simulink library "tqd"  (R2021b)
settings: Solver=VariableStepAuto  StartTime=0.0  StopTime=10.0  RelTol=1e-3
undefined symbols (not defined in the file or in its folder): ATQD_APSDecReq_X_kph, ATQD_APSDecReq_Y_mps2, ATQD_APSDecReqCMD_X_kph, ATQD_APSDecReqTs_X_pct, ATQD_APSDecTimeGain_X_Deg, ATQD_APSDecTimeGain_Y_s, ATQD_APSReqLowSpd_X_Deg, ATQD_AutoHoldReleaseBPS_X_Deg, ATQD_AWDLoadTrqnsGain_X_kg, ATQD_AWDLoadTrqnsGain_Y_pct, ATQD_BOSEnBPSPosn_X_kph, ATQD_BOSMap_X_rpm, ATQD_BOSMap_Y_pct, ATQD_CreepBaseTqD_X_kph, ATQD_CreepBaseTqD_Y_Deg, ATQD_CreepBaseTqR_X_kph, ATQD_CreepBaseTqR_Y_Deg, ATQD_CreepBPSDisPosn_X_Deg, ATQD_CreepBPSDisPosnR_X_Deg, ATQD_CreepBPSEnPosn_X_Deg, ATQD_CreepBPSEnPosnR_X_Deg, ATQD_CreepDeltaTq_X_kph, ATQD_CreepIterm_X_kph, ATQD_CreepIterm_Y_kph, ATQD_CreepItermMaxLimit_X_pct, ATQD_CreepPreloadTime_X_kph, ATQD_CreepPreloadTq_X_kph, ATQD_CreepPreloadTq_Y_s, ATQD_CreepProtTq_X_Deg, ATQD_CreepPterm_X_kph, ATQD_CreepPterm_Y_kph, ATQD_ECOTqMapD_X_rpm, ATQD_ECOTqMapD_Y_pct, ATQD_EOPDTqMapDCon_X_rpm, ATQD_EOPDTqMapDCon_Y_Deg, ATQD_EstInitVehWeight_X_c, ATQD_LHMRollGenMapD_X_rpm, ATQD_LHMRollGenMapD_Y_rpm, ATQD_LHMTqMapD_X_rpm, ATQD_LHMTqMapD_Y_pct, ATQD_NL1TqMapD_X_rpm, ATQD_NL1TqMapD_Y_pct, ATQD_NOPDTqMapDCon_X_rpm, ATQD_NOPDTqMapDCon_Y_Deg, ATQD_NRMRrEDUSpRat_X_rpm, ATQD_NRMRrEDUSpRat_Y_Nm, ATQD_OPDHoldDownRelDelay_X_Deg, ATQD_OPDHoldEnSpd_X_Deg, ATQD_OPDHoldRelDetTime_X_Deg, ATQD_OPDHoldReleaseTq_X_Deg, ATQD_OrigPedTqLowLim_X_Deg, ATQD_OrigPedTqLowLim_Y_pct, ATQD_PedalMapClimbUpLim_X_rpm, ATQD_PedalMapClimbUpLim_Y_Deg, ATQD_PreLoadTq_X_s, ATQD_RollGenMapEL1_X_rpm, ATQD_RollGenMapEL1_Y_rpm, ATQD_SL1TqMapD_X_rpm, ATQD_SL1TqMapD_Y_pct, ATQD_SlideRegenTqGain_X_Gps ... (+487)
libraries: hcu_lib x83, simulink x73, tqr x1
(part 12 of 19)

== system tqd/TQD/TorqueDemand/TorqueModule/OPD Hold/Parking Requeest Backup ==
  VTQD_APSReq_enum : Inport
  VTQD_APSReqTimer_s : Inport  Port=2
  VTQD_ParkRequest_flg : Inport  Port=3
  task_time_s : Inport  Port=4
  VTQD_AutiHoldRelease_flg : Inport  Port=5
  AND : Logic  AllPortsSameDT=off  OutDataTypeStr=boolean
  AND1 : Logic  AllPortsSameDT=off  OutDataTypeStr=boolean
  AND3 : Logic  Inputs=3  AllPortsSameDT=off  OutDataTypeStr=boolean
  Constant1 : Constant  Value=KTQD_APSReqDelayTime_s
  Constant16 : Constant  OutDataTypeStr=uint8
  Constant17 : Constant  Value=TRUE  OutDataTypeStr=uint8
  Constant2 : Constant  Value=KTQD_APSReqDelayTime_s
  Constant3 : Constant  Value=KTQD_OPDHoldBrkSW_flg
  Constant4 : Constant  Value=KTQD_OPDHoldAllowPark_flg
  Constant5 : Constant  Value=KTQD_OPDHoldAllowPark_s
  Constant6 : Constant  Value=KTQD_OPDHoldAllowGearPSW_flg
  DelayEnable : hcu_lib/Basic_Blocks/DelayEnable
  Equal6 : RelationalOperator  Operator===  OutDataTypeStr=boolean  RndMeth=Simplest
  NOT : Logic  Operator=NOT  AllPortsSameDT=off  OutDataTypeStr=boolean
  OR : Logic  Operator=OR  AllPortsSameDT=off  OutDataTypeStr=boolean
  Relational Operator1 : RelationalOperator  OutDataTypeStr=boolean  RndMeth=Simplest
  Relational Operator6 : RelationalOperator  OutDataTypeStr=boolean  RndMeth=Simplest
  SR_Latch : hcu_lib/Basic_Blocks/SR_Latch
  Switch4 : Switch  Criteria=u2 > Threshold
  VTQD_ActParkRequest_flg : Outport
  VTQD_OPDHoldAllowPark_flg : Outport  Port=2
  wires:
  Constant3/1 -> AND3/2
  Constant1/1 -> Relational Operator6/2
  Equal6/1 -> AND3/1
  [VTQD_APSReq_enum] -> Equal6/1
  Relational Operator6/1 -> AND3/3
  [VTQD_ParkRequest_flg] -> Switch4/3
  Constant17/1 -> Switch4/1
  Constant16/1 -> Equal6/2
  Switch4/1 -> [VTQD_ActParkRequest_flg]  "VTQD_ActParkRequest_flg"
  [VTQD_APSReqTimer_s] -> Relational Operator6/1
  VTQD_APSReq_enum/1 -> [VTQD_APSReq_enum]
  VTQD_APSReqTimer_s/1 -> [VTQD_APSReqTimer_s]
  VTQD_ParkRequest_flg/1 -> [VTQD_ParkRequest_flg]
  [VTQD_ActParkRequest_flg] -> VTQD_ActParkRequest_flg/1
  Constant2/1 -> Relational Operator1/2
  [VTQD_APSReqTimer_s] -> Relational Operator1/1
  task_time_s/1 -> [task_time_s]
  AND/1 -> DelayEnable/1
  Relational Operator1/1 -> AND/1
  Constant4/1 -> AND/2
  Constant5/1 -> DelayEnable/2
  DelayEnable/1 -> SR_Latch/1
  [VTQD_AutiHoldRelease_flg] -> SR_Latch/2
  VTQD_AutiHoldRelease_flg/1 -> [VTQD_AutiHoldRelease_flg]
  SR_Latch/1 -> [VTQD_OPDHoldAllowPark_flg]  "VTQD_OPDHoldAllowPark_flg"
  OR/1 -> Switch4/2
  AND3/1 -> OR/1
  [task_time_s] -> DelayEnable/3
  [VTQD_OPDHoldAllowPark_flg] -> AND1/1
  AND1/1 -> OR/2
  NOT/1 -> AND1/2
  Constant6/1 -> NOT/1
  [VTQD_OPDHoldAllowPark_flg] -> VTQD_OPDHoldAllowPark_flg/1

== system tqd/TQD/TorqueDemand/TorqueModule/OPD Hold/Release Condition ==
  VVMC_EstSlope_Deg : Inport
  VTQD_VehActSpd_kph : Inport  Port=2
  VTQR_NoABSFEDUWhlTqReq_Nm : Inport  Port=3
  VTQR_NoABSREDUWhlTqReq_Nm : Inport  Port=4
  VTQD_ActBPSPosn_pct : Inport  Port=5
  task_time_s : Inport  Port=6
  VTQD_APSReqTimer_s : Inport  Port=7
  VTQD_LowIdleAccPedal_flg : Inport  Port=8
  VTQD_OPDHoldRgnOn2Off_flg : Inport  Port=9
  VTQD_ActAPSPosn_pct : Inport  Port=10
  VTQD_FrOPDHoldRelTqGain_Nm : Inport  Port=11
  VTQD_RrOPDHoldRelTqGain_Nm : Inport  Port=12
  AND : Logic  Inputs=3  AllPortsSameDT=off  OutDataTypeStr=boolean
  AND1 : Logic  AllPortsSameDT=off  OutDataTypeStr=boolean
  AND2 : Logic  AllPortsSameDT=off  OutDataTypeStr=boolean
  AND3 : Logic  AllPortsSameDT=off  OutDataTypeStr=boolean
  Add : Sum
  Add1 : Sum  Inputs=+-+
  Add6 : Sum
  Add7 : Sum
  Constant1 : Constant  Value=KTQD_APSRelDisTqDev_Nm
  Constant{5,10,23,30} (4 alike) : Constant  Value=ZERO_FLOAT
  Constant2 : Constant  Value=KTQD_OPDHoldDownEnTime_s
  Constant36 : Constant  Value=KTQD_OPDHoldRelDetSpd_kph
  Constant4 : Constant  Value=KTQD_OPDHoldRelTqGain_Nm
  Constant6 : Constant  Value=KTQD_OPDHoldDetRevSpd_kph
  Constant7 : Constant  Value=KTQD_OPDHoldLiftRevSpd_kph
  Constant8 : Constant  Value=KTQD_APSDecReqMaxTime_s
  Constant9 : Constant  Value=KTQD_OPDHoldRelTqGain_Nm
  Delay{,1..3} (4 alike) : Delay  DelayLength=1
  DelayEnable : hcu_lib/Basic_Blocks/DelayEnable
  DelayEnable1 : hcu_lib/Basic_Blocks/DelayEnable
  Detect Increase : simulink/Logic and Bit Operations/Detect Increase  vinit=0.0  OutDataTypeStr=boolean
  Detect Increase1 : simulink/Logic and Bit Operations/Detect Increase  vinit=0.0  OutDataTypeStr=boolean
  Detect Increase2 : simulink/Logic and Bit Operations/Detect Increase  vinit=0.0  OutDataTypeStr=boolean
  MTQD_AutoHoldReleaseBPS_Y_pct : Lookup_n-D  NumberOfTableDimensions=1  BreakpointsForDimension1=ATQD_AutoHoldReleaseBPS_X_Deg  Table=MTQD_AutoHoldReleaseBPS_Y_pct  InternalRulePriority=Speed  RndMeth=Simplest  InputSameDT=on
  MTQD_OPDHoldDownRelDelay_Y_s : Lookup_n-D  NumberOfTableDimensions=1  BreakpointsForDimension1=ATQD_OPDHoldDownRelDelay_X_Deg  Table=MTQD_OPDHoldDownRelDelay_Y_s  InternalRulePriority=Speed  RndMeth=Simplest  InputSameDT=on
  MTQD_OPDHoldRelDetTime_Y_s : Lookup_n-D  NumberOfTableDimensions=1  BreakpointsForDimension1=ATQD_OPDHoldRelDetTime_X_Deg  Table=MTQD_OPDHoldRelDetTime_Y_s  InternalRulePriority=Speed  RndMeth=Simplest  InputSameDT=on
  MTQD_OPDHoldReleaseTq_Y_Nm{,1..3} (4 alike) : Lookup_n-D  NumberOfTableDimensions=1  BreakpointsForDimension1=ATQD_OPDHoldReleaseTq_X_Deg  Table=MTQD_OPDHoldReleaseTq_Y_Nm  InternalRulePriority=Speed  RndMeth=Simplest  InputSameDT=on
  Max : MinMax  Function=max  Inputs=2
  Max1 : MinMax  Function=max  Inputs=2
  Max2 : MinMax  Function=max  Inputs=2
  NOT{,1..5} (6 alike) : Logic  Operator=NOT  AllPortsSameDT=off  OutDataTypeStr=boolean
  OR : Logic  Operator=OR  AllPortsSameDT=off  OutDataTypeStr=boolean
  OR1 : Logic  Operator=OR  AllPortsSameDT=off  OutDataTypeStr=boolean
  OR2 : Logic  Operator=OR  AllPortsSameDT=off  OutDataTypeStr=boolean
  OR3 : Logic  Operator=OR  Inputs=3  AllPortsSameDT=off  OutDataTypeStr=boolean
  Relational Operator : RelationalOperator  Operator=>  OutDataTypeStr=boolean  RndMeth=Simplest
  Relational Operator1 : RelationalOperator  Operator=<=  OutDataTypeStr=boolean  RndMeth=Simplest
  Relational Operator3 : RelationalOperator  Operator=<=  OutDataTypeStr=boolean  RndMeth=Simplest
  Relational Operator4 : RelationalOperator  OutDataTypeStr=boolean  RndMeth=Simplest
  Relational Operator5 : RelationalOperator  Operator=<  OutDataTypeStr=boolean  RndMeth=Simplest
  Relational Operator6 : RelationalOperator  Operator=>  OutDataTypeStr=boolean  RndMeth=Simplest
  Relational Operator7 : RelationalOperator  OutDataTypeStr=boolean  RndMeth=Simplest
  Relational Operator9 : RelationalOperator  OutDataTypeStr=boolean  RndMeth=Simplest
  Relay : Relay  OnSwitchValue=KTQD_OPDHoldGradeUp_Deg  OffSwitchValue=KTQD_OPDHoldGradeDown_Deg  OutDataTypeStr=boolean
  Relay1 : Relay  OnSwitchValue=KTQD_OPDHoldGradeUp_Deg  OffSwitchValue=KTQD_OPDHoldGradeDown_Deg  OutDataTypeStr=boolean
  SR_Latch : hcu_lib/Basic_Blocks/SR_Latch
  SR_Latch1 : hcu_lib/Basic_Blocks/SR_Latch
  Switch{,1..6} (7 alike) : Switch  Criteria=u2 > Threshold
  Terminator : Terminator
  VTQD_AutoHoldRelease_flg : Outport
  VTQD_OPDHoldEnRel_flg : Outport  Port=2
  VTQD_OPDHoldActRelTq_Nm : Outport  Port=3
  wires:
  VVMC_EstSlope_Deg/1 -> [VVMC_EstSlope_Deg]
  VTQD_VehActSpd_kph/1 -> [VTQD_VehActSpd_kph]
  VTQR_NoABSFEDUWhlTqReq_Nm/1 -> [VTQR_NoABSFEDUWhlTqReq_Nm]
  VTQR_NoABSREDUWhlTqReq_Nm/1 -> [VTQR_NoABSREDUWhlTqReq_Nm]
  VTQD_ActBPSPosn_pct/1 -> [VTQD_ActBPSPosn_pct]
  task_time_s/1 -> [task_time_s]
  [VTQD_AutoHoldRelease_flg] -> VTQD_AutoHoldRelease_flg/1
  [VTQD_OPDHoldEnRel_flg] -> VTQD_OPDHoldEnRel_flg/1
  VTQD_APSReqTimer_s/1 -> [VTQD_APSReqTimer_s]
  VTQD_LowIdleAccPedal_flg/1 -> [VTQD_LowIdleAccPedal_flg]
  VTQD_OPDHoldRgnOn2Off_flg/1 -> [VTQD_OPDHoldRgnOn2Off_flg]
  VTQD_ActAPSPosn_pct/1 -> Terminator/1
  VTQD_RrOPDHoldRelTqGain_Nm/1 -> [VTQD_RrOPDHoldRelTqGain_Nm]
  VTQD_FrOPDHoldRelTqGain_Nm/1 -> [VTQD_FrOPDHoldRelTqGain_Nm]
  SR_Latch/1 -> DelayEnable/1  "VTQD_OPDHoldEnRelLatch_flg"
  Detect Increase2/1 -> OR2/1
  Detect Increase1/1 -> SR_Latch1/1
  DelayEnable1/1 -> Switch1/1
  SR_Latch1/1 -> [VTQD_OPDHoldRelReverse_flg]  "VTQD_OPDHoldRelReverse_flg"
  MTQD_OPDHoldDownRelDelay_Y_s/1 -> [VTQD_OPDHoldDownRelDelay_s]  "VTQD_OPDHoldDownRelDelay_s"
  Constant4/1 -> Switch2/1
  [VVMC_EstSlope_Deg] -> MTQD_OPDHoldDownRelDelay_Y_s/1
  [task_time_s] -> DelayEnable1/3
  [VTQD_LowIdleAccPedal_flg] -> NOT2/1
  Constant30/1 -> Switch5/1
  NOT/1 -> AND/2
  [VVMC_EstSlope_Deg] -> Relay1/1
  Relay1/1 -> NOT3/1
  Constant2/1 -> Relational Operator1/2
  OR1/1 -> AND/3
  Switch1/1 -> Switch/3
  AND2/1 -> Switch1/3
  [VTQD_LowIdleAccPedal_flg] -> NOT1/1
  [VTQD_OPDHoldRgnOn2Off_flg] -> Switch/2
  Relational Operator/1 -> OR1/1
  Relational Operator1/1 -> AND/1
  [VTQD_OPDHoldRelDetTime_s] -> DelayEnable/2
  AND/1 -> OR/1
  [VVMC_EstSlope_Deg] -> Relay/1
  [VTQR_NoABSFEDUWhlTqReq_Nm] -> Add6/1
  [VTQR_NoABSREDUWhlTqReq_Nm] -> Add6/2
  [task_time_s] -> DelayEnable/3
  [VTQR_NoABSFEDUWhlTqReq_Nm] -> Add7/1
  [VTQD_ActBPSPosn_pct] -> Relational Operator/1
  Add1/1 -> Max1/1
  [VVMC_EstSlope_Deg] -> MTQD_OPDHoldReleaseTq_Y_Nm/1
  DelayEnable/1 -> [VTQD_OPDHoldEnRel_flg]  "VTQD_OPDHoldEnRel_flg"
  [VTQR_NoABSREDUWhlTqReq_Nm] -> Add7/2
  Max1/1 -> Relational Operator5/2
  [VTQD_VehActSpd_kph] -> Relational Operator9/1
  Relational Operator9/1 -> Switch5/2
  [VVMC_EstSlope_Deg] -> MTQD_AutoHoldReleaseBPS_Y_pct/1
  [VVMC_EstSlope_Deg] -> MTQD_OPDHoldRelDetTime_Y_s/1
  Switch5/1 -> [VTQD_OPDHoldRelDetTime_s]  "VTQD_OPDHoldRelDetTime_s"
  MTQD_AutoHoldReleaseBPS_Y_pct/1 -> Relational Operator/2  "VTQD_AutoHoldReleaseAPS_pct"
  OR/1 -> [VTQD_AutoHoldRelease_flg]  "VTQD_AutoHoldRelease_flg"
  MTQD_OPDHoldReleaseTq_Y_Nm/1 -> Switch6/3
  Relational Operator3/1 -> Detect Increase1/1
  [VTQD_OPDHoldDownRelDelay_s] -> DelayEnable1/2
  Delay3/1 -> Max2/1
  Max2/1 -> Switch6/1
  Constant6/1 -> Relational Operator3/2
  Detect Increase/1 -> OR3/1
  Add7/1 -> Relational Operator5/1  "VTQD_OPDHoldDisRelTq_Nm"
  Switch6/1 -> Add/2, Delay3/1  "VTQD_OPDHoldReleaseTq_Nm"
  [VVMC_EstSlope_Deg] -> MTQD_OPDHoldReleaseTq_Y_Nm3/1
  [VTQD_APSReqTimer_s] -> Delay/1
  NOT3/1 -> Switch1/2
  [VTQD_OPDHoldRelReverse_flg] -> Detect Increase2/1
  [VTQD_OPDHoldRelReverse_flg] -> Switch6/2
  Constant23/1 -> Max1/2
  [VTQD_LowIdleAccPedal_flg] -> NOT4/1
  MTQD_OPDHoldRelDetTime_Y_s/1 -> Switch5/3
  [VTQD_OPDHoldRelReverse_flg] -> Switch3/2
  Relational Operator4/1 -> SR_Latch/1  "VTQD_OPDHoldEnRelease_flg"
  Switch2/1 -> Add/1
  NOT5/1 -> AND2/2
  MTQD_OPDHoldReleaseTq_Y_Nm1/1 -> Switch4/3
  Relay/1 -> NOT/1
  Add/1 -> [VTQD_OPDHoldActRelTq_Nm], Relational Operator4/2  "VTQD_OPDHoldActRelTq_Nm"
  [VTQD_OPDHoldRelReverse_flg] -> Switch4/2
  Delay/1 -> Relational Operator1/1
  Constant8/1 -> Relational Operator7/2
  OR2/1 -> SR_Latch/2
  [VTQD_VehActSpd_kph] -> Relational Operator3/1
  Delay2/1 -> Max/1
  [VTQD_OPDHoldEnRel_flg] -> AND1/2
  AND1/1 -> Switch/1
  [VTQD_LowIdleAccPedal_flg] -> AND3/1
  [VTQD_LowIdleAccPedal_flg] -> NOT5/1
  Constant36/1 -> Relational Operator9/2
  NOT4/1 -> DelayEnable1/1
  [VTQD_APSReqTimer_s] -> Delay1/1
  Constant10/1 -> Switch3/3
  MTQD_OPDHoldReleaseTq_Y_Nm2/1 -> Max/2
  [VTQD_LowIdleAccPedal_flg] -> Detect Increase/1
  Add6/1 -> Relational Operator4/1  "VTQD_OPDHoldEnRelTq_flg"
  [VTQD_OPDHoldRelReverse_flg] -> Switch2/2
  Switch3/1 -> Add1/1
  [VVMC_EstSlope_Deg] -> MTQD_OPDHoldReleaseTq_Y_Nm1/1
  Relational Operator5/1 -> OR2/2  "VTQD_OPDHoldDisRelease_flg"
  MTQD_OPDHoldReleaseTq_Y_Nm3/1 -> Max2/2
  Delay1/1 -> Relational Operator7/1
  Relational Operator7/1 -> AND3/2
  Constant7/1 -> Relational Operator6/2
  Switch4/1 -> Delay2/1, Add1/3
  Constant5/1 -> Switch2/3
  AND3/1 -> OR3/3
  Constant9/1 -> Switch3/1
  Switch/1 -> OR/2
  NOT2/1 -> AND1/1
  [VTQD_VehActSpd_kph] -> Relational Operator6/1
  [VTQD_OPDHoldEnRel_flg] -> AND2/1
  Constant1/1 -> Add1/2
  NOT1/1 -> OR1/2
  Relational Operator6/1 -> OR3/2
  Max/1 -> Switch4/1
  [VVMC_EstSlope_Deg] -> MTQD_OPDHoldReleaseTq_Y_Nm2/1
  OR3/1 -> SR_Latch1/2
  [VTQD_OPDHoldActRelTq_Nm] -> VTQD_OPDHoldActRelTq_Nm/1

== system tqd/TQD/TorqueDemand/TorqueModule/OPD Hold/System Status ==
  VTQD_GearActualPosn_enum : Inport
  VINP_EPBSta_enum : Inport  Port=2
  VTQD_RegenMode_enum : Inport  Port=3
  VTQD_AutiHoldRelease_flg : Inport  Port=4
  VTQD_AntiBlockRrActDisTime_s : Inport  Port=5
  VTQD_RrAntiBlockAactive_flg : Inport  Port=6
  VTQD_ActBPSPosn_pct : Inport  Port=7
  VTQD_AntiBlockFrActDisTime_s : Inport  Port=8
  VTQD_FrAntiBlockAactive_flg : Inport  Port=9
  VVMC_ADASActive_flg : Inport  Port=10
  VPMM_PwrSta_enum : Inport  Port=11
  VVMC_CruzActive_flg : Inport  Port=12
  VTQD_VehActSpd_kph : Inport  Port=13
  VVMC_EstSlope_Deg : Inport  Port=14
  task_time_s : Inport  Port=15
  VINP_FrPTCSActive_flg : Inport  Port=16
  VINP_RrPTCSActive_flg : Inport  Port=17
  VINP_ESCActive_flg : Inport  Port=18
  VINP_ABSActive_flg : Inport  Port=19
  VVMC_APSActive_flg : Inport  Port=20
  AND{,3..6} (5 alike) : Logic  AllPortsSameDT=off  OutDataTypeStr=boolean
  AND1 : Logic  Inputs=4  AllPortsSameDT=off  OutDataTypeStr=boolean
  AND2 : Logic  Inputs=11  AllPortsSameDT=off  OutDataTypeStr=boolean
  Constant1 : Constant  Value=2  OutDataTypeStr=uint8
  Constant10 : Constant  Value=ENUM_GEARACTUALPOSN_R
  Constant11 : Constant  Value=ENUM_GEARACTUALPOSN_D
  Constant12 : Constant  Value=KTQD_R2DGradeUpLim_Deg
  Constant13 : Constant  Value=KTQD_R2DGradeLowLim_Deg
  Constant14 : Constant  Value=KTQD_R2DEnOPDHoldSpd_kph
  Constant15 : Constant  Value=KTQD_R2DEnOPDHSpdDelayTime_s
  Constant2 : Constant  Value=0  OutDataTypeStr=uint8
  Constant3 : Constant  Value=ENUM_EPBSTA_APPLIED
  Constant4 : Constant  Value=ENUM_GEARACTUALPOSN_P
  Constant40 : Constant  Value=ENUM_REGENLEVEL_OPD
  Constant44 : Constant  Value=ENUM_REGENLEVEL_OPD
  Constant45 : Constant  Value=ENUM_POWERSTA_READY
  Constant5 : Constant  Value=ENUM_GEARACTUALPOSN_D
  Constant6 : Constant  Value=KTQD_AutoHoldEnSpd_kph
  Constant7 : Constant  Value=ENUM_EPBSTA_APPLIED
  Constant8 : Constant  Value=ENUM_REGENLEVEL_OPD
  Constant9 : Constant  Value=ENUM_GEARACTUALPOSN_P
  Delay : Delay  DelayLength=1
  Delay2 : Delay  DelayLength=1
  Delay3 : Delay  DelayLength=1
  DelayEnable : hcu_lib/Basic_Blocks/DelayEnable
  Equal{1..2,5..6,8..9,11,30} (8 alike) : RelationalOperator  Operator===  OutDataTypeStr=boolean  RndMeth=Simplest
  Equal10 : RelationalOperator  Operator=~=  OutDataTypeStr=boolean  RndMeth=Simplest
  Equal3 : RelationalOperator  Operator=~=  OutDataTypeStr=boolean  RndMeth=Simplest
  Equal4 : RelationalOperator  Operator=~=  OutDataTypeStr=boolean  RndMeth=Simplest
  GreaterThan3 : RelationalOperator  Operator=>  OutDataTypeStr=boolean  RndMeth=Simplest
  NOT{,1..7} (8 alike) : Logic  Operator=NOT  AllPortsSameDT=off  OutDataTypeStr=boolean
  OR : Logic  Operator=OR  AllPortsSameDT=off  OutDataTypeStr=boolean
  OR1 : Logic  Operator=OR  AllPortsSameDT=off  OutDataTypeStr=boolean
  OR5 : Logic  Operator=OR  AllPortsSameDT=off  OutDataTypeStr=boolean
  Relational Operator : RelationalOperator  Operator=<=  OutDataTypeStr=boolean  RndMeth=Simplest
  Relational Operator1 : RelationalOperator  OutDataTypeStr=boolean  RndMeth=Simplest
  Relational Operator2 : RelationalOperator  OutDataTypeStr=boolean  RndMeth=Simplest
  Relational Operator3 : RelationalOperator  Operator=<=  OutDataTypeStr=boolean  RndMeth=Simplest
  SR_Latch3 : hcu_lib/Basic_Blocks/SR_Latch
  SR_Latch4 : hcu_lib/Basic_Blocks/SR_Latch
  Switch : Switch  Criteria=u2 > Threshold
  Unit Delay1 : UnitDelay  SampleTime=-1  HasFrameUpgradeWarning=on
  VTQD_APSStaSys_enum : Outport
  VTQD_OPDHoldDelayForP_flg : Outport  Port=2
  VTQD_OPDHoldRgnOn2Off_flg : Outport  Port=3
  wires:
  Switch/1 -> [VTQD_APSStaSys_enum]  "VTQD_APSStaSys_enum"
  Constant2/1 -> Switch/3
  AND2/1 -> Switch/2
  Constant1/1 -> Switch/1
  [VTQD_GearActualPosn_enum] -> Equal1/1
  Equal1/1 -> AND5/1
  AND5/1 -> [VTQD_OPDHoldDelayForP_flg]  "VTQD_OPDHoldDelayForP_flg"
  Equal10/1 -> AND5/2
  [VTQD_RegenMode_enum] -> Equal8/1
  OR5/1 -> [VTQD_AntiBlockEnOPDHold_flg]  "VTQD_AntiBlockEnOPDHold_flg"
  Equal8/1 -> OR5/2
  Constant40/1 -> Equal8/2
  Equal11/1 -> GreaterThan3/2, Unit Delay1/1
  SR_Latch3/1 -> [VTQD_OPDHoldRgnOn2Off_flg]  "VTQD_OPDHoldRgnOn2Off_flg"
  GreaterThan3/1 -> AND6/2
  Constant45/1 -> Equal30/2
  AND6/1 -> SR_Latch3/1
  [VPMM_PwrSta_enum] -> Equal30/1
  Equal30/1 -> AND6/1
  Unit Delay1/1 -> GreaterThan3/1
  [VTQD_AutiHoldRelease_flg] -> Delay/1
  Constant44/1 -> Equal11/2
  [VTQD_RegenMode_enum] -> Equal11/1
  Constant3/1 -> Equal10/2
  [VINP_EPBSta_enum] -> Equal10/1
  Constant4/1 -> Equal1/2
  [VTQD_OPDHoldRgnOn2Off_flg] -> OR5/1
  VTQD_GearActualPosn_enum/1 -> [VTQD_GearActualPosn_enum]
  VINP_EPBSta_enum/1 -> [VINP_EPBSta_enum]
  VTQD_RegenMode_enum/1 -> [VTQD_RegenMode_enum]
  VTQD_AutiHoldRelease_flg/1 -> [VTQD_AutiHoldRelease_flg]
  VTQD_AntiBlockRrActDisTime_s/1 -> [VTQD_AntiBlockRrActDisTime_s]
  VTQD_RrAntiBlockAactive_flg/1 -> [VTQD_RrAntiBlockAactive_flg]
  VTQD_ActBPSPosn_pct/1 -> [VTQD_ActBPSPosn_pct]
  VTQD_AntiBlockFrActDisTime_s/1 -> [VTQD_AntiBlockFrActDisTime_s]
  VTQD_FrAntiBlockAactive_flg/1 -> [VTQD_FrAntiBlockAactive_flg]
  VVMC_ADASActive_flg/1 -> [VVMC_ADASActive_flg]
  VPMM_PwrSta_enum/1 -> [VPMM_PwrSta_enum]
  VVMC_CruzActive_flg/1 -> [VVMC_CruzActive_flg]
  VTQD_VehActSpd_kph/1 -> [VTQD_VehActSpd_kph]
  [VTQD_APSStaSys_enum] -> VTQD_APSStaSys_enum/1
  [VTQD_OPDHoldDelayForP_flg] -> VTQD_OPDHoldDelayForP_flg/1
  [VTQD_OPDHoldRgnOn2Off_flg] -> VTQD_OPDHoldRgnOn2Off_flg/1
  Constant9/1 -> Equal5/2
  Equal4/1 -> AND/1
  [VTQD_GearActualPosn_enum] -> Equal5/1
  Constant8/1 -> Equal4/2
  AND/1 -> OR/2
  [VTQD_RegenMode_enum] -> Equal4/1
  Equal5/1 -> AND/2
  Delay/1 -> OR/1
  OR/1 -> SR_Latch3/2
  Delay2/1 -> Equal6/1
  Constant12/1 -> Relational Operator/2
  [VTQD_OPDHoldR2D_flg] -> Delay3/1
  Constant13/1 -> Relational Operator1/2
  DelayEnable/1 -> SR_Latch4/2  "VTQD_R2DEnOPDHold_flg"
  [VVMC_EstSlope_Deg] -> Relational Operator1/1
  [task_time_s] -> DelayEnable/3
  [VTQD_GearActualPosn_enum] -> Delay2/1
  Constant11/1 -> Equal9/2
  [VTQD_GearActualPosn_enum] -> Equal9/1
  Constant14/1 -> Relational Operator2/2
  [VTQD_VehActSpd_kph] -> Relational Operator2/1
  AND4/1 -> DelayEnable/1
  Constant10/1 -> Equal6/2
  Relational Operator1/1 -> AND1/4
  AND1/1 -> SR_Latch4/1
  Relational Operator/1 -> AND1/3
  Constant15/1 -> DelayEnable/2
  Delay3/1 -> AND4/1
  [VVMC_EstSlope_Deg] -> Relational Operator/1
  Equal6/1 -> AND1/1
  SR_Latch4/1 -> [VTQD_OPDHoldR2D_flg]  "VTQD_OPDHoldR2D_flg"
  Equal9/1 -> AND1/2
  Relational Operator2/1 -> AND4/2
  [VTQD_VehActSpd_kph] -> Relational Operator3/1
  Relational Operator3/1 -> AND2/5
  OR1/1 -> AND2/3
  Constant6/1 -> Relational Operator3/2
  Equal3/1 -> AND2/6
  NOT3/1 -> AND2/1
  NOT4/1 -> AND2/4
  [VINP_ABSActive_flg] -> NOT6/1
  NOT6/1 -> AND2/10
  NOT1/1 -> AND2/7
  [VINP_ESCActive_flg] -> NOT5/1
  [VINP_EPBSta_enum] -> Equal3/1
  Constant7/1 -> Equal3/2
  NOT5/1 -> AND2/9
  NOT2/1 -> AND2/8
  [VINP_RrPTCSActive_flg] -> NOT2/1
  [VVMC_CruzActive_flg] -> NOT4/1
  AND3/1 -> OR1/1
  Equal2/1 -> AND3/1
  [VTQD_GearActualPosn_enum] -> Equal2/1
  NOT/1 -> AND3/2
  [VTQD_OPDHoldR2D_flg] -> NOT/1
  Constant5/1 -> Equal2/2
  [VTQD_AntiBlockEnOPDHold_flg] -> AND2/2
  [VTQD_OPDHoldDelayForP_flg] -> OR1/2
  [VVMC_ADASActive_flg] -> NOT3/1
  [VINP_FrPTCSActive_flg] -> NOT1/1
  VVMC_EstSlope_Deg/1 -> [VVMC_EstSlope_Deg]
  task_time_s/1 -> [task_time_s]
  VINP_ABSActive_flg/1 -> [VINP_ABSActive_flg]
  VINP_FrPTCSActive_flg/1 -> [VINP_FrPTCSActive_flg]
  VINP_ESCActive_flg/1 -> [VINP_ESCActive_flg]
  VINP_RrPTCSActive_flg/1 -> [VINP_RrPTCSActive_flg]
  NOT7/1 -> AND2/11
  [VVMC_APSActive_flg] -> NOT7/1
  VVMC_APSActive_flg/1 -> [VVMC_APSActive_flg]

== system tqd/TQD/TorqueDemand/TorqueModule/TqCoordination/Coordinate_ADAS ==
  VVMC_ADASWhlTqReq_Nm : Inport
  VTQD_PreLoadHold_flg : Inport  Port=2
  VTQD_DriverWhlTqDem_Nm : Inport  Port=3
  Action Port : ActionPort  ActionPortLabel=elseif( u3 ~= 0)
  Constant9 : Constant  Value=ENUM_TQSOURCE_ADAS
  Switch : Switch  Criteria=u2 > Threshold
  VTQD_ADASWhlTqReq_Nm : Outport
  VTQD_TqSourceADAS_enum : Outport  Port=2
  wires:
  VTQD_DriverWhlTqDem_Nm/1 -> Switch/1
  Switch/1 -> VTQD_ADASWhlTqReq_Nm/1
  VTQD_PreLoadHold_flg/1 -> Switch/2
  Constant9/1 -> VTQD_TqSourceADAS_enum/1
  VVMC_ADASWhlTqReq_Nm/1 -> Switch/3

== system tqd/TQD/TorqueDemand/TorqueModule/TqCoordination/Coordinate_ADASForceIdle ==
  Action Port : ActionPort  ActionPortLabel=elseif(u2 ~= 0)
  Constant : Constant  Value=ZERO_FLOAT
  Constant8 : Constant  Value=ENUM_TQSOURCE_ADASFORCEIDLE
  VTQD_ADASForceIdleReq_Nm : Outport
  VTQD_ADASForceIdle_enum : Outport  Port=2
  wires:
  Constant8/1 -> VTQD_ADASForceIdle_enum/1
  Constant/1 -> VTQD_ADASForceIdleReq_Nm/1

== system tqd/TQD/TorqueDemand/TorqueModule/TqCoordination/Coordinate_APS ==
  VTQD_DriverWhlTqDem_Nm : Inport
  Action Port : ActionPort  ActionPortLabel=elseif( u6 ~= 0)
  Constant9 : Constant  Value=ENUM_TQSOURCE_APS
  VTQD_APSWhlTqReq_Nm : Outport
  VTQD_TqSourceAPS_enum : Outport  Port=2
  wires:
  Constant9/1 -> VTQD_TqSourceAPS_enum/1
  VTQD_DriverWhlTqDem_Nm/1 -> VTQD_APSWhlTqReq_Nm/1

== system tqd/TQD/TorqueDemand/TorqueModule/TqCoordination/Coordinate_Cruise ==
  VVMC_CruzWhlTqReq_Nm : Inport
  Action Port : ActionPort  ActionPortLabel=elseif( u4 ~= 0)
  Constant9 : Constant  Value=ENUM_TQSOURCE_CC
  VTQD_CruzWhlTqReq_Nm : Outport
  VTQD_TqSourceCruz_enum : Outport  Port=2
  wires:
  Constant9/1 -> VTQD_TqSourceCruz_enum/1
  VVMC_CruzWhlTqReq_Nm/1 -> VTQD_CruzWhlTqReq_Nm/1

== system tqd/TQD/TorqueDemand/TorqueModule/TqCoordination/Coordinate_DirverPedal ==
  VTQD_DriverWhlTqDem_Nm : Inport
  Action Port : ActionPort  ActionPortLabel=else
  Constant9 : Constant  Value=ENUM_TQSOURCE_INTERNAL
  VTQD_DriverWhlTqReq_Nm : Outport
  VTQD_TqSourceInternal_enum : Outport  Port=2
  wires:
  VTQD_DriverWhlTqDem_Nm/1 -> VTQD_DriverWhlTqReq_Nm/1
  Constant9/1 -> VTQD_TqSourceInternal_enum/1

== system tqd/TQD/TorqueDemand/TorqueModule/TqCoordination/Coordinate_MSA ==
  VVMC_MSAWhlTqReq_Nm : Inport
  Action Port : ActionPort  ActionPortLabel=elseif( u5 ~= 0)
  Constant9 : Constant  Value=ENUM_TQSOURCE_MSA
  VTQD_MSAWhlTqReq_Nm : Outport
  VTQD_TqSourceMSA_enum : Outport  Port=2
  wires:
  Constant9/1 -> VTQD_TqSourceMSA_enum/1
  VVMC_MSAWhlTqReq_Nm/1 -> VTQD_MSAWhlTqReq_Nm/1

== system tqd/TQD/TorqueDemand/TorqueModule/TqCoordination/Coordinate_NoSuitbleGear_flg ==
  Action Port : ActionPort
  Constant5 : Constant  Value=KTQD_DriverTqDemN_Nm
  Constant8 : Constant  Value=ENUM_TQSOURCE_INVALID
  VTQD_GearNoSuitReq_Nm : Outport
  VTQD_TqSourceGearNoSuit_enum : Outport  Port=2
  wires:
  Constant5/1 -> VTQD_GearNoSuitReq_Nm/1
  Constant8/1 -> VTQD_TqSourceGearNoSuit_enum/1

== system tqd/TQD/TorqueDemand/TorqueModule/TqDistribution/AWD_Ratio ==
  note: initia:2000kg
  VTQD_DriverWhlTqDem_Nm : Inport
  VTQD_RrShaftSpd_rpm : Inport  Port=2
  VTQD_EVDriveMode_enum : Inport  Port=3
  VTQD_LimpHomeAct_flg : Inport  Port=4
  VVMC_APSActive_flg : Inport  Port=5
  VTQD_CreepPrLoadEnable_flg : Inport  Port=6
  VTQD_EstVehWeightResult_kg : Inport  Port=7
  VVMC_ActLRSlideRate_pct : Inport  Port=8
  VVMC_ActRRSlideRate_pct : Inport  Port=9
  VVMC_RearTqRatio_rat : Inport  Port=10
  Action Port : ActionPort
  AND : Logic  AllPortsSameDT=off  OutDataTypeStr=boolean
  Abs : Abs
  Abs1 : Abs
  Constant : Constant  Value=ONE_FLOAT
  Constant1 : Constant  Value=ONE_FLOAT
  Constant10 : Constant  Value=KTQD_AWDRrRatio_rat_ovrdflg  VectorParams1D=off  SampleTime=-1
  Constant11 : Constant  Value=KTQD_AWDRrRatio_rat_ovrdval  VectorParams1D=off  SampleTime=-1
  Constant12 : Constant  Value=KTQD_DrvSelPwrTrainSW_flg  VectorParams1D=off  SampleTime=-1
  Constant13 : Constant  Value=KTQD_AWDWhlTqRatioSW_flg
  Constant14 : Constant  Value=KTQD_WhlRatioDisCreep_flg
  Constant2 : Constant  Value=ENUM_DRIVEMODE_ECO
  Constant3 : Constant  Value=ENUM_DRIVETRAIN_FWD  VectorParams1D=off  SampleTime=-1
  Constant4 : Constant  Value=ENUM_DRIVETRAIN_AWD  VectorParams1D=off  SampleTime=-1
  Constant5 : Constant  Value=ENUM_DRIVEMODE_SPORT
  Constant6 : Constant  Value=ZERO_FLOAT
  Constant7 : Constant  Value=ONE_FLOAT
  Constant8 : Constant  Value=KTQD_AWDFrRatio_rat_ovrdflg  VectorParams1D=off  SampleTime=-1
  Constant9 : Constant  Value=KTQD_AWDFrRatio_rat_ovrdval  VectorParams1D=off  SampleTime=-1
  Equal : RelationalOperator  Operator===  OutDataTypeStr=boolean  RndMeth=Simplest
  Equal1 : RelationalOperator  Operator=~=  OutDataTypeStr=boolean  RndMeth=Simplest
  Equal2 : RelationalOperator  Operator===  OutDataTypeStr=boolean  RndMeth=Simplest
  Equal3 : RelationalOperator  Operator===  OutDataTypeStr=boolean  RndMeth=Simplest
  Ground : Ground
  LiuzgSwitch{1..5,13} (6 alike) : Switch  Criteria=u2 ~= 0
      settings: AttributesFormatString=<%<Criteria>>
  MTQD_AWDLoadTrqnsGain_Z_c : Lookup_n-D  BreakpointsForDimension1=ATQD_AWDLoadTrqnsGain_Y_pct  BreakpointsForDimension2=ATQD_AWDLoadTrqnsGain_X_kg  Table=MTQD_AWDLoadTrqnsGain_Z_c  ExtrapMethod=Clip  InternalRulePriority=Speed  RndMeth=Simplest  InputSameDT=on
      settings: InputPortMap=u0,u1
  MTQD_ECORrEDUSpRat_Z_rat : Lookup_n-D  BreakpointsForDimension1=ATQD_NRMRrEDUSpRat_Y_Nm  BreakpointsForDimension2=ATQD_NRMRrEDUSpRat_X_rpm  Table=MTQD_ECORrEDUSpRat_Z_rat  ExtrapMethod=Clip  InternalRulePriority=Speed  RndMeth=Simplest  InputSameDT=on
      settings: InputPortMap=u0,u1
  "MTQD_NRMRrEDUSpRat_Z_rat  " : Lookup_n-D  BreakpointsForDimension1=ATQD_NRMRrEDUSpRat_Y_Nm  BreakpointsForDimension2=ATQD_NRMRrEDUSpRat_X_rpm  Table=MTQD_NRMRrEDUSpRat_Z_rat  ExtrapMethod=Clip  InternalRulePriority=Speed  RndMeth=Simplest  InputSameDT=on
      settings: InputPortMap=u0,u1
  "MTQD_SPORTRrEDUSpRat_Z_rat " : Lookup_n-D  BreakpointsForDimension1=ATQD_NRMRrEDUSpRat_Y_Nm  BreakpointsForDimension2=ATQD_NRMRrEDUSpRat_X_rpm  Table=MTQD_SPORTRrEDUSpRat_Z_rat  ExtrapMethod=Clip  InternalRulePriority=Speed  RndMeth=Simplest  InputSameDT=on
      settings: InputPortMap=u0,u1
  Max : MinMax  Function=max  Inputs=2
  NOT : Logic  Operator=NOT  AllPortsSameDT=off  OutDataTypeStr=boolean
  OR : Logic  Operator=OR  AllPortsSameDT=off  OutDataTypeStr=boolean
  OR1 : Logic  AllPortsSameDT=off  OutDataTypeStr=boolean
  Product : Product
  Saturation : Saturate  UpperLimit=KTQD_RrEDUTqDistrictMax_gain  LowerLimit=KTQD_RrEDUTqDistrictMin_gain
      settings: AttributesFormatString=|
      | <%<UpperLimit>>
      | <%<LowerLimit>>
  Subtract : Sum  Inputs=+-
  Switch : Switch  Criteria=u2 > Threshold
  Switch1 : Switch  Criteria=u2 > Threshold
  Switch2 : Switch  Criteria=u2 > Threshold
  VTQD_FrRatio_AWD : Outport
  VTQD_RrRatio_AWD : Outport  Port=2
  wires:
  Constant/1 -> Subtract/1
  Saturation/1 -> Switch1/3, Subtract/2
  VTQD_EVDriveMode_enum/1 -> [VTQD_EVDriveMode_enum]
  VTQD_DriverWhlTqDem_Nm/1 -> [VTQD_DriverWhlTqDem_Nm]
  VTQD_RrShaftSpd_rpm/1 -> [VTQD_RrShaftSpd_rpm]
  [VTQD_DriverWhlTqDem_Nm] -> "MTQD_NRMRrEDUSpRat_Z_rat  "/1
  [VTQD_RrShaftSpd_rpm] -> "MTQD_NRMRrEDUSpRat_Z_rat  "/2
  VTQD_LimpHomeAct_flg/1 -> [VTQD_LimpHomeAct_flg]
  [VTQD_LimpHomeAct_flg] -> LiuzgSwitch13/2
  Equal/1 -> LiuzgSwitch1/2
  "MTQD_SPORTRrEDUSpRat_Z_rat "/1 -> LiuzgSwitch1/1
  [VTQD_EVDriveMode_enum] -> Equal/1
  Constant5/1 -> Equal/2
  [VTQD_DriverWhlTqDem_Nm] -> "MTQD_SPORTRrEDUSpRat_Z_rat "/1
  [VTQD_RrShaftSpd_rpm] -> "MTQD_SPORTRrEDUSpRat_Z_rat "/2
  "MTQD_NRMRrEDUSpRat_Z_rat  "/1 -> LiuzgSwitch1/3, LiuzgSwitch13/1
  [VTQD_RrShaftSpd_rpm] -> MTQD_ECORrEDUSpRat_Z_rat/2
  [VTQD_DriverWhlTqDem_Nm] -> MTQD_ECORrEDUSpRat_Z_rat/1
  Constant2/1 -> Equal2/2
  [VTQD_EVDriveMode_enum] -> Equal2/1
  MTQD_ECORrEDUSpRat_Z_rat/1 -> LiuzgSwitch3/1
  Equal2/1 -> LiuzgSwitch3/2
  LiuzgSwitch3/1 -> LiuzgSwitch13/3
  LiuzgSwitch1/1 -> LiuzgSwitch3/3
  OR/1 -> OR1/1
  [VTQD_CreepPrLoadEnable_flg] -> OR/2
  Constant1/1 -> LiuzgSwitch2/1
  [VVMC_APSActive_flg] -> OR/1
  VVMC_APSActive_flg/1 -> [VVMC_APSActive_flg]
  VTQD_CreepPrLoadEnable_flg/1 -> [VTQD_CreepPrLoadEnable_flg]
  Product/1 -> Switch2/3
  LiuzgSwitch13/1 -> Product/1
  MTQD_AWDLoadTrqnsGain_Z_c/1 -> [VTQD_AWDLoadTrqnsGain_c]  "VTQD_AWDLoadTrqnsGain_c"
  [VTQD_AWDLoadTrqnsGain_c] -> Product/2
  VTQD_EstVehWeightResult_kg/1 -> [VTQD_EstVehWeightResult_kg]
  [VTQD_EstVehWeightResult_kg] -> MTQD_AWDLoadTrqnsGain_Z_c/2
  LiuzgSwitch2/1 -> LiuzgSwitch4/3
  [VINP_DriverSelPowerTrain_enum] -> Equal1/1
  Constant4/1 -> Equal1/2
  LiuzgSwitch5/1 -> LiuzgSwitch4/1
  Constant3/1 -> Equal3/2
  [VINP_DriverSelPowerTrain_enum] -> Equal3/1
  Equal3/1 -> LiuzgSwitch5/2
  LiuzgSwitch4/1 -> Saturation/1
  Constant7/1 -> LiuzgSwitch5/3
  Constant6/1 -> LiuzgSwitch5/1
  Ground/1 -> [VINP_DriverSelPowerTrain_enum]  "VINP_DriverSelPowerTrain_enum"
  Subtract/1 -> Switch/3
  Switch/1 -> VTQD_FrRatio_AWD/1  "VTQD_FrEDUSpRat_rat"
  Switch1/1 -> VTQD_RrRatio_AWD/1  "VTQD_RrEDUSpRat_rat"
  Constant8/1 -> Switch/2
  Constant9/1 -> Switch/1
  Constant11/1 -> Switch1/1
  Constant10/1 -> Switch1/2
  Constant12/1 -> AND/2
  Equal1/1 -> AND/1
  AND/1 -> LiuzgSwitch4/2
  VVMC_ActRRSlideRate_pct/1 -> [VVMC_ActRRSlideRate_pct]
  VVMC_ActLRSlideRate_pct/1 -> [VVMC_ActLRSlideRate_pct]
  [VVMC_ActLRSlideRate_pct] -> Abs/1
  [VVMC_ActRRSlideRate_pct] -> Abs1/1
  Abs1/1 -> Max/2
  Abs/1 -> Max/1
  Max/1 -> MTQD_AWDLoadTrqnsGain_Z_c/1  "VTQD_AWDLoadTrqnsGain_pct"
  Constant13/1 -> Switch2/2
  VVMC_RearTqRatio_rat/1 -> Switch2/1
  Switch2/1 -> LiuzgSwitch2/3
  OR1/1 -> LiuzgSwitch2/2
  Constant14/1 -> NOT/1
  NOT/1 -> OR1/2

== system tqd/TQD/TorqueDemand/TorqueModule/TqDistribution/FWD_Ratio ==
  Action Port : ActionPort
  Constant : Constant  Value=ONE_FLOAT
  Constant1 : Constant  Value=ZERO_FLOAT
  VTQD_FrRatio_FWD : Outport
  VTQD_RrRatio_FWD : Outport  Port=2
  wires:
  Constant/1 -> VTQD_FrRatio_FWD/1
  Constant1/1 -> VTQD_RrRatio_FWD/1

== system tqd/TQD/TorqueDemand/TorqueModule/TqDistribution/RWD_Ratio ==
  Action Port : ActionPort
  Constant : Constant  Value=ONE_FLOAT
  Constant1 : Constant  Value=ZERO_FLOAT
  VTQD_FrRatio_RWD : Outport
  VTQD_RrRatio_RWD : Outport  Port=2
  wires:
  Constant1/1 -> VTQD_FrRatio_RWD/1
  Constant/1 -> VTQD_RrRatio_RWD/1

== system tqd/TQD/TorqueDemand/Signal_convert/SWC2_Subsystem/Speed Setting Mode/ACC Speed Setting ON ==
  note: Old ACC Set Speed
  note: ACCSetSpd_241018
  note: ACC SPEED SETTING Signal
  VTQD_SWC2ScrollUpSta_enum : Inport
  VTQD_SWC2ScrollDownSta_enum : Inport  Port=2
  task_time_s : Inport  Port=3
  VVMC_LVDAACCStatusInformation_flg : Inport  Port=4
  VVMC_ACCObjDist_m : Inport  Port=5
  VTQD_SpdLim4SetSpd_raw32 : Inport  Port=6
  VINP_ADASACCSta_enum : Inport  Port=7
  VINP_Distanceunit_flg : Inport  Port=8
  VTQD_SWC2ResUpSta_flg : Inport  Port=9
  VTQD_SWC2SetDownSta_flg : Inport  Port=10
  VINP_SmartEcoModeSW_flg : Inport  Port=11
  VVMC_SetACCDisableAPS_flg : Inport  Port=12
  VINP_IVIACCAdaptiveSta_flg : Inport  Port=13
  VTQD_Set2MeterSpd_flg : Inport  Port=14
  VTQD_SetRoadSpdLim_flg : Inport  Port=15
  VINP_ADASSLIFSpdLim_enum : Inport  Port=16
  VTQD_LScrollPressShort_flg : Inport  Port=17
  VVMC_MeterIndSpeed_raw32 : Inport  Port=18
  Action Port : ActionPort  InitializeStates=reset
  " 20" : Constant  Value=KTQD_ACCActiveMetSpdLoMPH_mph
  " 30kph" : Constant  Value=KTQD_ACCActiveMetSpdLo_kph
  0 : Constant  Value=KTQD_AllowSetSpdOvrd_flg
  1 : Constant  Value=KTQD_AllowSetSpdOvrdVal_flg
  105 : Constant  Value=KTQD_ACCActiveMetSpdHiMPH_mph
  10kph1 : Constant  Value=KTQD_AllowSetSpdSpd_kph
  180kph : Constant  Value=KTQD_ACCActiveMetSpdHi_kph
  2 : Constant  Value=KTQD_SmartEcoLimitSpd_kph
  2m : Constant  Value=KVMC_NotAllowSetSpdDist_m
  3 : Constant  Value=KTQD_SmartEcoLimitSpd_mph
  5 : Constant  Value=KTQD_SetSpdDeltaLongMPH_mph
  5kph : Constant  Value=KTQD_SetSpdDeltaLong_kph
  6m : Constant  Value=KVMC_AllowSetSpdDist_m
  ACCSetSpd_241018 : Stateflow chart  TreatAsAtomicUnit=on
  ACCSetSpd_Chart_W : Stateflow chart  TreatAsAtomicUnit=on
      settings: PortSchema="{\"entries\":[{\"content\":{\"sides\":[{\"content\":{\"connectorIds\":[\"In1\",\"In2\",\"In3\",\"In4\",\"In5\",\"In6\",\"In7\",\"In8\",\"In11\",\"In12\",\"In13\",\"In9\",\"In10\"]},\"type\":\"ConnectorPlacement.EquallySpacedRectSide\",\"uuid\":\"61ce72b2-2f56-4065-9e06-1345412a8c86\"},{\"content\":{\"connectorIds\":[\"Out1\"],\"side\":\"RIGHT\"},\"type\":\"ConnectorPlacement.EquallySpacedRectSide\",\"uuid\":\"4594d6d3-f7cd-4711-8df0-9a0a2c5601b5\"},{\"content\":{\"connectorIds\":[],\"side\":\"TOP\"},\"type\":\"ConnectorPlacement.EquallySpacedRectSide\",\"uuid\":\"a8857ab2-f9b0-4737-b2f3-522f42c1ada3\"}]},\"type\":\"ConnectorPlacement.EquallySpacedConnector\",\"uuid\":\"0a7f8e6a-9c19-454d-bd26-d3d8923cc49e\"}],\"packageUris\":[\"http://schema.mathworks.com/mf0/Connector/R2020b\"],\"version\":\"1.0\"}"
  AND : Logic  AllPortsSameDT=off  OutDataTypeStr=boolean
  AND1 : Logic  AllPortsSameDT=off  OutDataTypeStr=boolean
  AND2 : Logic  AllPortsSameDT=off  OutDataTypeStr=boolean
  Cast To Single : DataTypeConversion  OutDataTypeStr=int8
  Constant126 : Constant  Value=0x0  OutDataTypeStr=uint8
  Equal53 : RelationalOperator  Operator=~=  OutDataTypeStr=boolean  RndMeth=Simplest
  ONE : Constant  Value=ONE_INT
  OR : Logic  Operator=OR  AllPortsSameDT=off  OutDataTypeStr=boolean
  Relational Operator : RelationalOperator  Operator=<=  OutDataTypeStr=boolean  RndMeth=Simplest
  Relational Operator1 : RelationalOperator  Operator=>  OutDataTypeStr=boolean  RndMeth=Simplest
  Relational Operator2 : RelationalOperator  Operator===  OutDataTypeStr=boolean  RndMeth=Simplest
  Relational Operator3 : RelationalOperator  OutDataTypeStr=boolean  RndMeth=Simplest
  Relational Operator4 : RelationalOperator  Operator===  OutDataTypeStr=boolean  RndMeth=Simplest
  Round : Rounding  Operator=round
  Switch{,1..7} (8 alike) : Switch  Criteria=u2 > Threshold
  standby : Constant  Value=ENUM_ADASACCSTA_STANDBY
  standby1 : Constant  Value=KTQD_ACCSetSpdSource_flg
  zero : Constant  Value=ZERO_INT
  VTQD_ACCSetSpd_kph : Outport
  VTQD_SWC2AllowSetSpd_flg : Outport  Port=2
  wires:
  VVMC_LVDAACCStatusInformation_flg/1 -> [VVMC_LVDAACCStatusInformation_flg]
  task_time_s/1 -> [task_time_s]
  Switch4/1 -> [VTQD_SetSpdDeltaLong_raw32]  "VTQD_SetSpdDeltaLong_raw32"
  Switch3/1 -> [VTQD_ACCActiveMetSpdLo_raw32]  "VTQD_ACCActiveMetSpdLo_raw32"
  VTQD_SpdLim4SetSpd_raw32/1 -> [VTQD_SpdLim4SetSpd_raw32]
  VINP_ADASACCSta_enum/1 -> [VINP_ADASACCSta_enum]
  6m/1 -> Relational Operator/2
  2m/1 -> Relational Operator1/2
  Relational Operator/1 -> AND/1
  Relational Operator1/1 -> AND/2
  [VTQD_SpdLim4SetSpd_raw32] -> Relational Operator3/1
  10kph1/1 -> Relational Operator3/2
  AND/1 -> OR/1
  Relational Operator3/1 -> OR/2
  Switch/1 -> VTQD_SWC2AllowSetSpd_flg/1, [VTQD_AllowSetSpd_flg]  "VTQD_SWC2AllowSetSpd_flg"
  OR/1 -> AND2/1
  0/1 -> Switch/2
  1/1 -> Switch/1
  Cast To Single/1 -> Relational Operator4/1, Switch1/3
  Switch1/1 -> VTQD_ACCSetSpd_kph/1
  [VINP_ADASACCSta_enum] -> Relational Operator2/1
  AND1/1 -> Switch1/2
  ONE/1 -> Switch1/1
  standby/1 -> Relational Operator2/2
  zero/1 -> Relational Operator4/2
  Relational Operator2/1 -> AND1/1
  Relational Operator4/1 -> AND1/2
  VINP_Distanceunit_flg/1 -> [VINP_Distanceunit_flg]
  [VINP_Distanceunit_flg] -> Switch2/2
  Switch2/1 -> [VTQD_ACCActiveMetSpdHi_raw32]  "VTQD_ACCActiveMetSpdHi_raw32"
  [VINP_Distanceunit_flg] -> Switch3/2
  " 30kph"/1 -> Switch3/3
  " 20"/1 -> Switch3/1
  [VINP_Distanceunit_flg] -> Switch4/2
  5kph/1 -> Switch4/3
  5/1 -> Switch4/1
  Round/1 -> Cast To Single/1
  VTQD_SWC2ScrollUpSta_enum/1 -> [VTQD_SWC2ScrollUpSta_enum]
  VTQD_SWC2SetDownSta_flg/1 -> [VTQD_SWC2SetDownSta_flg]
  VTQD_SWC2ResUpSta_flg/1 -> [VTQD_SWC2ResUpSta_flg]
  VINP_SmartEcoModeSW_flg/1 -> [VINP_SmartEcoModeSW_flg]
  180kph/1 -> Switch5/3
  [VINP_SmartEcoModeSW_flg] -> Switch5/2
  Switch5/1 -> Switch2/3
  [VINP_SmartEcoModeSW_flg] -> Switch6/2
  105/1 -> Switch6/3
  Switch6/1 -> Switch2/1
  3/1 -> Switch6/1
  2/1 -> Switch5/1
  AND2/1 -> Switch/3
  [VINP_ADASACCSta_enum] -> ACCSetSpd_241018/1(VINP_ADASACCSta_enum)
  [VTQD_SpdLim4SetSpd_raw32] -> ACCSetSpd_241018/3(VTQD_SpdLim4SetSpd_raw32)
  [VTQD_ACCActiveMetSpdHi_raw32] -> ACCSetSpd_241018/4(VTQD_ACCActiveMetSpdHi_raw32)
  [VTQD_ACCActiveMetSpdLo_raw32] -> ACCSetSpd_241018/5(VTQD_ACCActiveMetSpdLo_raw32)
  [VTQD_SWC2ScrollUpSta_enum] -> ACCSetSpd_241018/7(VTQD_SWC2ScrollUpSta_enum)
  [VTQD_SWC2ScrollDownSta_enum] -> ACCSetSpd_241018/8(VTQD_SWC2ScrollDownSta_enum)
  [VTQD_SetSpdDeltaLong_raw32] -> ACCSetSpd_241018/9(VTQD_SetSpdDeltaLong_raw32)
  [VINP_Distanceunit_flg] -> ACCSetSpd_241018/11(VINP_Distanceunit_flg)
  Constant126/1 -> Equal53/2
  ACCSetSpd_241018/1(VTQD_ACCSetSpd_raw32) -> [VTQD_ACCSetSpd_raw32]  "VTQD_ACCSetSpd_raw32"
  Switch7/1 -> Round/1
  [VTQD_ACCSetSpd_raw32] -> Switch7/1
  standby1/1 -> Switch7/2
  [VVMC_LVDAACCStatusInformation_flg] -> ACCSetSpd_241018/14(VVMC_LVDAACCStatusInformation_flg)
  VTQD_SWC2ScrollDownSta_enum/1 -> [VTQD_SWC2ScrollDownSta_enum]
  VVMC_ACCObjDist_m/1 -> [VVMC_ACCObjDist_m]
  [VVMC_ACCObjDist_m] -> Relational Operator/1
  [VVMC_ACCObjDist_m] -> Relational Operator1/1
  VVMC_SetACCDisableAPS_flg/1 -> [VVMC_SetACCDisableAPS_flg]
  [VVMC_SetACCDisableAPS_flg] -> AND2/2
  VINP_IVIACCAdaptiveSta_flg/1 -> [VINP_IVIACCAdaptiveSta_flg]
  [VINP_IVIACCAdaptiveSta_flg] -> ACCSetSpd_241018/2(VINP_IVIACCAdaptiveSta_flg)
  VTQD_Set2MeterSpd_flg/1 -> [VTQD_Set2MeterSpd_flg]
  [VTQD_Set2MeterSpd_flg] -> ACCSetSpd_241018/6(VTQD_Set2MeterSpd_flg)
  VTQD_SetRoadSpdLim_flg/1 -> [VTQD_SetRoadSpdLim_flg]
  [VTQD_SetRoadSpdLim_flg] -> ACCSetSpd_241018/10(VTQD_SetRoadSpdLim_flg)
  VINP_ADASSLIFSpdLim_enum/1 -> [VINP_ADASSLIFSpdLim_enum]
  [VINP_ADASSLIFSpdLim_enum] -> Equal53/1
  VTQD_LScrollPressShort_flg/1 -> [VTQD_LScrollPressShort_flg]
  [VTQD_LScrollPressShort_flg] -> ACCSetSpd_241018/13(VTQD_LScrollPressShort_flg)
  VVMC_MeterIndSpeed_raw32/1 -> [VVMC_MeterIndSpeed_raw32]
  [VVMC_MeterIndSpeed_raw32] -> ACCSetSpd_241018/15(VVMC_MeterIndSpeed_raw32)
  Equal53/1 -> [VTQD_ADASSLIFSpdLimDet_flg]  "VTQD_ADASSLIFSpdLimDet_flg"
  [VTQD_ADASSLIFSpdLimDet_flg] -> ACCSetSpd_241018/12(VTQD_ADASSLIFSpdLimDet_flg)
  [VINP_ADASACCSta_enum] -> ACCSetSpd_Chart_W/1(VINP_ADASACCSta_enum)
  [VTQD_SWC2ResUpSta_flg] -> ACCSetSpd_Chart_W/2(VTQD_SWC2ResUpSta_flg)
  [VTQD_SWC2SetDownSta_flg] -> ACCSetSpd_Chart_W/3(VTQD_SWC2SetDownSta_flg)
  [VTQD_SpdLim4SetSpd_raw32] -> ACCSetSpd_Chart_W/4(VVMC_MeterIndSpeed_raw32)
  [VTQD_ACCActiveMetSpdHi_raw32] -> ACCSetSpd_Chart_W/5(KTQD_ACCActiveMetSpdHi_raw32)
  [VINP_Distanceunit_flg] -> ACCSetSpd_Chart_W/6(VINP_Distanceunit_flg)
  [VTQD_ACCActiveMetSpdLo_raw32] -> ACCSetSpd_Chart_W/7(KTQD_ACCActiveMetSpdLo_raw32)
  [VTQD_SetSpdDeltaLong_raw32] -> ACCSetSpd_Chart_W/8(KTQD_SetSpdDeltaLong_kph)
  [task_time_s] -> ACCSetSpd_Chart_W/11(task_time_s)
  [VTQD_SWC2ScrollUpSta_enum] -> ACCSetSpd_Chart_W/12(VTQD_SWC2ScrollUpSta_enum)
  [VTQD_SWC2ScrollDownSta_enum] -> ACCSetSpd_Chart_W/13(VTQD_SWC2ScrollDownSta_enum)
  [VVMC_LVDAACCStatusInformation_flg] -> ACCSetSpd_Chart_W/9(VVMC_LVDAACCStatusInformation_flg)
  [VTQD_AllowSetSpd_flg] -> ACCSetSpd_Chart_W/10(VTQD_AllowSetSpd_flg)
  ACCSetSpd_Chart_W/1(VTQD_ACCSetSpd_kph) -> [VTQD_ACCSetSpd_kph]  "VTQD_ACCSetSpd_kph"
  [VTQD_ACCSetSpd_kph] -> Switch7/3

== system tqd/TQD/TorqueDemand/Signal_convert/SWC2_Subsystem/Speed Setting Mode/CC Speed Setting ON ==
  note: CC SPEED SETTING MODE
  VVMC_CCCtrlSta_enum : Inport
  "VTQD_SWCResUpPress_enum  " : Inport  Port=2
  "VTQD_SWCSetDownPress_enum  " : Inport  Port=3
  VTQD_SpdLim4SetSpd_raw32 : Inport  Port=4
  VTQD_SetSpdDeltaLongFit_kph : Inport  Port=5
  VINP_Distanceunit_flg : Inport  Port=6
  VINP_SmartEcoModeSW_flg : Inport  Port=7
  Action Port : ActionPort  InitializeStates=reset
  " 1" : Constant  Value=KTQD_CCActiveMetSpdLo_kph
  " 2" : Constant  Value=KTQD_CCActiveMetSpdLoMPH_mph
  1 : Constant  Value=KTQD_SetSpdDeltaLongFit_kph
  2 : Constant  Value=KTQD_SetSpdDeltaShort_kph
  3 : Constant  Value=KTQD_CCActiveMetSpdHi_kph
  4 : Constant  Value=KTQD_SetSpdDeltaLong_kph
  5 : Constant  Value=KTQD_CCActiveMetSpdHiMPH_mph
  6 : Constant  Value=KTQD_SetSpdDeltaLongMPH_mph
  7 : Constant  Value=KTQD_SmartEcoLimitSpd_kph
  8 : Constant  Value=KTQD_SmartEcoLimitSpd_mph
  AND1 : Logic  AllPortsSameDT=off  OutDataTypeStr=boolean
  CC Speed Setting Mode : Stateflow chart  TreatAsAtomicUnit=on
      settings: PortSchema="{\"entries\":[{\"content\":{\"sides\":[{\"content\":{\"connectorIds\":[\"In5\",\"In12\",\"In4\",\"In3\",\"In9\",\"In6\",\"In7\",\"In8\",\"In1\",\"In2\",\"In11\",\"In10\"]},\"type\":\"ConnectorPlacement.EquallySpacedRectSide\",\"uuid\":\"331c8dfa-4564-419d-9323-fdbf8561d50b\"},{\"content\":{\"connectorIds\":[\"Out1\",\"Out2\"],\"side\":\"RIGHT\"},\"type\":\"ConnectorPlacement.EquallySpacedRectSide\",\"uuid\":\"71cb1444-7708-4b6f-91dd-d8a1c8c14ea8\"},{\"content\":{\"connectorIds\":[],\"side\":\"TOP\"},\"type\":\"ConnectorPlacement.EquallySpacedRectSide\",\"uuid\":\"6ecf38bb-d171-491a-a8b2-073f135e7039\"}]},\"type\":\"ConnectorPlacement.EquallySpacedConnector\",\"uuid\":\"fc3afa97-6e6e-4933-9aff-7c8f8cbb1702\"}],\"packageUris\":[\"http://schema.mathworks.com/mf0/Connector/R2020b\"],\"version\":\"1.0\"}"
  Cast To Single : DataTypeConversion  OutDataTypeStr=int8
  ONE : Constant  Value=ONE_INT
  Relational Operator2 : RelationalOperator  Operator===  OutDataTypeStr=boolean  RndMeth=Simplest
  Relational Operator4 : RelationalOperator  Operator===  OutDataTypeStr=boolean  RndMeth=Simplest
  Round : Rounding  Operator=round
  Specific_STATE_ChangeToSTANDBY : Stateflow chart  TreatAsAtomicUnit=on
  Switch{,1..5} (6 alike) : Switch  Criteria=u2 > Threshold
  standby : Constant  Value=ENUM_ADASCCSTA_STANDBY
  zero : Constant  Value=ZERO_INT
  VTQD_CCSetSpd_kph : Outport
  VTQD_SWC2CCSpdResetFinish_flg : Outport  Port=2
  wires:
  "VTQD_SWCSetDownPress_enum  "/1 -> CC Speed Setting Mode/10(VTQD_SWCSetDownPress_enum)
  [VTQD_ChangeToSTANDBY_flg] -> CC Speed Setting Mode/12(VTQD_ChangeToSTANDBY_flg)
  Specific_STATE_ChangeToSTANDBY/1(VTQD_CCChangeToSTANDBY_flg) -> [VTQD_ChangeToSTANDBY_flg]
  [VVMC_CCCtrlSta_enum] -> Specific_STATE_ChangeToSTANDBY/1(VVMC_CCCtrlSta_enum)
  "VTQD_SWCResUpPress_enum  "/1 -> CC Speed Setting Mode/11(VTQD_SWCResUpPress_enum)
  VVMC_CCCtrlSta_enum/1 -> CC Speed Setting Mode/5(VVMC_CCCtrlSta_enum), [VVMC_CCCtrlSta_enum]
  Switch2/1 -> CC Speed Setting Mode/7(KTQD_CCActiveMetSpdHi_raw32)
  2/1 -> CC Speed Setting Mode/2(KTQD_SetSpdDeltaShort_kph)
  Switch3/1 -> CC Speed Setting Mode/8(KTQD_CCActiveMetSpdLo_raw32)
  Switch4/1 -> CC Speed Setting Mode/1(KTQD_SetSpdDeltaLong_kph)
  CC Speed Setting Mode/2(VTQD_CCSpdResetFinish_flg) -> VTQD_SWC2CCSpdResetFinish_flg/1  "VTQD_SWC2CCSpdResetFinish_flg"
  VTQD_SetSpdDeltaLongFit_kph/1 -> CC Speed Setting Mode/4(VTQD_SetSpdDeltaLongFit_kph)
  1/1 -> CC Speed Setting Mode/3(KTQD_SetSpdDeltaLongFit_kph)
  VTQD_SpdLim4SetSpd_raw32/1 -> CC Speed Setting Mode/9(VVMC_MeterIndSpeed_raw32)
  Cast To Single/1 -> Relational Operator4/1, Switch1/3
  Switch1/1 -> VTQD_CCSetSpd_kph/1
  [VVMC_CCCtrlSta_enum] -> Relational Operator2/1
  AND1/1 -> Switch1/2
  ONE/1 -> Switch1/1
  standby/1 -> Relational Operator2/2
  zero/1 -> Relational Operator4/2
  Relational Operator2/1 -> AND1/1
  Relational Operator4/1 -> AND1/2
  [VINP_Distanceunit_flg] -> Switch2/2
  VINP_Distanceunit_flg/1 -> [VINP_Distanceunit_flg]
  [VINP_Distanceunit_flg] -> Switch3/2
  " 1"/1 -> Switch3/3
  " 2"/1 -> Switch3/1
  [VINP_Distanceunit_flg] -> Switch4/2
  4/1 -> Switch4/3
  6/1 -> Switch4/1
  [VINP_Distanceunit_flg] -> CC Speed Setting Mode/6(VINP_Distanceunit_flg)
  Round/1 -> Cast To Single/1
  CC Speed Setting Mode/1(VTQD_CCSetSpd_kph) -> Round/1
  VINP_SmartEcoModeSW_flg/1 -> [VINP_SmartEcoModeSW_flg]
  [VINP_SmartEcoModeSW_flg] -> Switch/2
  3/1 -> Switch/3
  Switch/1 -> Switch2/3
  5/1 -> Switch5/3
  [VINP_SmartEcoModeSW_flg] -> Switch5/2
  Switch5/1 -> Switch2/1
  8/1 -> Switch5/1
  7/1 -> Switch/1

== system tqd/TQD/TorqueDemand/Signal_convert/SWC2_Subsystem/Speed Setting Mode/Else Speed Setting On ==
  In : Inport
  Action Port : ActionPort
  Data Type Conversion : DataTypeConversion
  Out : Outport
  wires:
  Data Type Conversion/1 -> Out/1
  In/1 -> Data Type Conversion/1

== system tqd/TQD/TorqueDemand/Signal_convert/SWC2_Subsystem/Speed Setting Mode/ISA Speed Setting ON ==
  VINP_ADASSLIFSpdLim_enum : Inport
  VINP_SmartEcoModeSW_flg : Inport  Port=2
  Action Port : ActionPort
  8 : Constant  Value=KTQD_SmartEcoLimitSpd_kph
  Data Type Conversion : DataTypeConversion
  Min : MinMax  Inputs=2
  Switch : Switch  Criteria=u2 > Threshold
  VTQD_ISASetSpd_kph : Outport
  wires:
  Data Type Conversion/1 -> VTQD_ISASetSpd_kph/1
  VINP_SmartEcoModeSW_flg/1 -> Switch/2
  VINP_ADASSLIFSpdLim_enum/1 -> Min/2, Switch/3
  Min/1 -> Switch/1
  8/1 -> Min/1
  Switch/1 -> Data Type Conversion/1
